simulink model "laba4_Guassian_Filter"  (Simulink 7.5)
settings: Solver=ode45  StartTime=0.0  StopTime=10.0  RelTol=1e-3
undefined symbols (not defined in the file): Fs, get, sided, Two
libraries: commfilt2 x4, commrandsrc2 x1, dspsnks4 x1, commutil2 x1
settings Model: Creator=Lenovo  LastModifiedBy=Lenovo

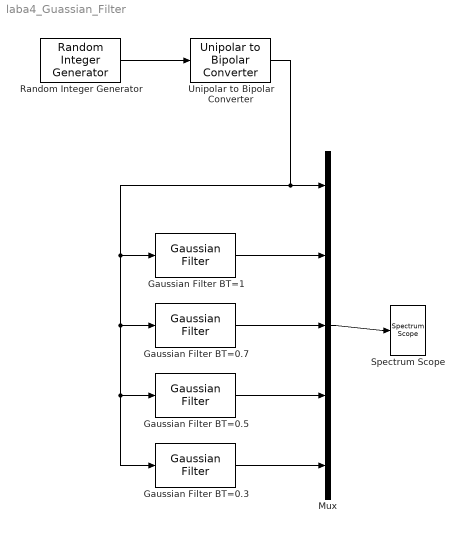
== system laba4_Guassian_Filter ==
  Gaussian Filter BT=0.3 : commfilt2/Gaussian Filter  DialogController=dspDDGCreate  DialogControllerArgs=DataTag0  SystemSampleTime=-1  N=8  BT=0.3  D=2  sampMode=Frame-based  normMode=Sum of coefficients  filterGain=1  checkCoeff=off  variableName=gaussFilt  launchFVT=off  roundingMode=Floor  overflowMode=off
  Gaussian Filter BT=0.5 : commfilt2/Gaussian Filter  DialogController=dspDDGCreate  DialogControllerArgs=DataTag1  SystemSampleTime=-1  N=8  BT=0.5  D=2  sampMode=Frame-based  normMode=Sum of coefficients  filterGain=1  checkCoeff=off  variableName=gaussFilt  launchFVT=off  roundingMode=Floor  overflowMode=off
  Gaussian Filter BT=0.7 : commfilt2/Gaussian Filter  DialogController=dspDDGCreate  DialogControllerArgs=DataTag2  SystemSampleTime=-1  N=8  BT=0.7  D=2  sampMode=Frame-based  normMode=Sum of coefficients  filterGain=1  checkCoeff=off  variableName=gaussFilt  launchFVT=off  roundingMode=Floor  overflowMode=off
  Gaussian Filter BT=1 : commfilt2/Gaussian Filter  DialogController=dspDDGCreate  DialogControllerArgs=DataTag3  SystemSampleTime=-1  N=8  BT=1  D=2  sampMode=Frame-based  normMode=Sum of coefficients  filterGain=1  checkCoeff=off  variableName=gaussFilt  launchFVT=off  roundingMode=Floor  overflowMode=off
  Mux : Mux  Inputs=5
  Random Integer Generator : commrandsrc2/Random Integer Generator  SystemSampleTime=-1  mul=2  seed=500  Ts=1/270000  frameBased=off  sampPerFrame=1  orient=off  outDataType=double
  Spectrum Scope : dspsnks4/Spectrum Scope  DialogController=dspdialog.SpectrumScope  DialogControllerArgs=DataTag4  SystemSampleTime=-1  ScopeProperties=on  Domain=Frequency  HorizSpan=1  UseBuffer=off  BufferSize=128  Overlap=64  inpFftLenInherit=off  FFTlength=128  numAvg=2  DisplayProperties=off  AxisGrid=on  Memory=off  FrameNumber=on  AxisLegend=off  AxisZoom=off  OpenScopeAtSimStart=on  OpenScopeImmediately=off  FigPos=get(0,'defaultfigureposition')  AxisProperties=off  XUnits=Hertz  XRange=Two-sided ((-Fs/2...Fs/2])  XDisplay=0  InheritXIncr=on  XIncr=1.0  XLabel=Samples  XLimit=Auto  YUnits=dBW/Hertz  XMax=1  XMin=0  YLabel=Magnitude-squared, dB  LineProperties=off  wintypeSpecScope=Hann  RsSpecScope=50  betaSpecScope=5  winsampSpecScope=Periodic  XAxisParamsVer=6.9
      settings: YMin=-10  YMax=10
  Unipolar to Bipolar Converter : commutil2/Unipolar to Bipolar Converter  SystemSampleTime=-1  M=2  polarity=Positive  dataType=Inherit via internal rule
  wires:
  Random Integer Generator/1 -> Unipolar to Bipolar Converter/1
  Mux/1 -> Spectrum Scope/1
  Gaussian Filter BT=0.3/1 -> Mux/5
  Gaussian Filter BT=0.5/1 -> Mux/4
  Gaussian Filter BT=0.7/1 -> Mux/3
  Gaussian Filter BT=1/1 -> Mux/2
  Unipolar to Bipolar Converter/1 -> Mux/1, Gaussian Filter BT=1/1, Gaussian Filter BT=0.7/1, Gaussian Filter BT=0.5/1, Gaussian Filter BT=0.3/1
